simulink model "Reto1y2"  (R2013a)
settings: Solver=ode45  StartTime=0.0  StopTime=10.0  RelTol=1e-3
values from neighbouring files (symbols this model uses):
  L = length(h)    [Reto4.m]
undefined symbols (not defined in the file or in its folder): C, R
settings Model: Creator=Henry Orlando  LastModifiedBy=Henry Orlando

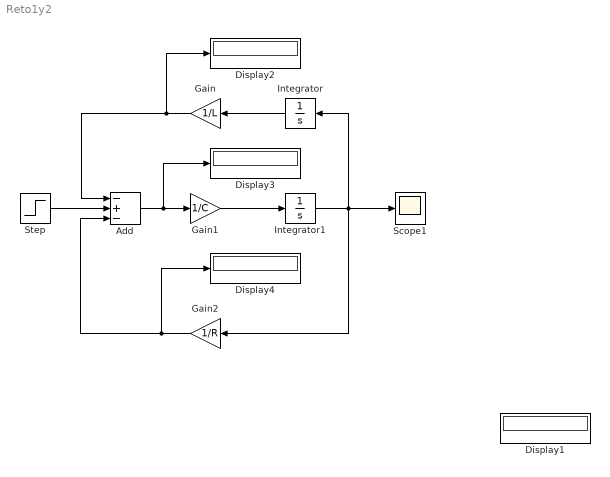
== system Reto1y2 ==
  Add : Sum  Inputs=-+-
  Display{1..4} (4 alike) : Display
  Gain : Gain  Gain=1/L
  Gain1 : Gain  Gain=1/C
  Gain2 : Gain  Gain=1/R
  Integrator : Integrator  InitialCondition=0.5
  Integrator1 : Integrator  InitialCondition=0.5
  Scope1 : Scope
  Step : Step  Time=5  Before=10  After=30  SampleTime=0
  wires:
  Step/1 -> Add/2
  Add/1 -> Display3/1, Gain1/1
  Gain2/1 -> Display4/1, Add/3
  Gain/1 -> Display2/1, Add/1
  Gain1/1 -> Integrator1/1
  Integrator/1 -> Gain/1
  Integrator1/1 -> Gain2/1, Integrator/1, Scope1/1
